simulink model "Linear_Control_Lab_Lab6_ServoMotor_Position_Control_1"  (R2018b)
settings: Solver=VariableStepAuto  StartTime=0.0  StopTime=30.0  RelTol=1e-3
settings Model: Creator=HP  LastModifiedBy=HP

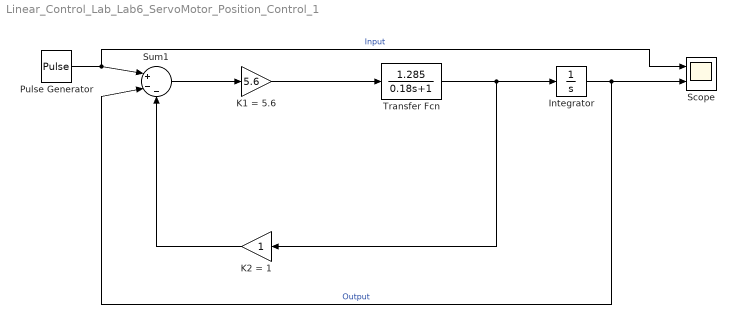
== system Linear_Control_Lab_Lab6_ServoMotor_Position_Control_1 ==
  Integrator : Integrator
  K1 = 5.6 : Gain  Gain=5.6
  K2 = 1 : Gain
  Pulse Generator : DiscretePulseGenerator  PulseType=Time based  Amplitude=3  Period=10  PulseWidth=50
  Scope : Scope  NumInputPorts=2
  Sum1 : Sum  Inputs=|+--
  Transfer Fcn : TransferFcn  Numerator=[1.285]  Denominator=[0.18 1]
  wires:
  Transfer Fcn/1 -> K2 = 1/1, Integrator/1
  K1 = 5.6/1 -> Transfer Fcn/1
  Sum1/1 -> K1 = 5.6/1
  Pulse Generator/1 -> Scope/1, Sum1/1  "Input"
  Integrator/1 -> Scope/2, Sum1/2  "Output"
  K2 = 1/1 -> Sum1/3
